simulink model "pipeline_13bit"  (R2022b)
settings: Solver=FixedStepDiscrete  StartTime=0.0  StopTime=5000*ts  FixedStep=ts  RelTol=1e-3
values from neighbouring files (symbols this model uses):
  beta = 1.01    [ADC_13bit.m]
  bits_number = 13    [ADC_13bit.m]
  C = 10e-12    (= 1e-11)    [ADC_13bit.m]
  fin = antismear(fin_pre,fs,nfft)    [ADC_13bit.m]
  Gain = 5000    [ADC_13bit.m]
  k = 1.380649e-23    [ADC_13bit.m]
  T = 300    [ADC_13bit.m]
  ts = 1/fs    (= 1)    [ADC_13bit.m]
(part 3 of 3)

== system pipeline_13bit/SHA_less_13_bit/Subsystem/stage_1p5_bit7/Comparator 2 ==
  Vin : Inport
  Vref : Inport  Port=2
  Output 1 or 0 : Relay  OnSwitchValue=0  OffSwitchValue=0
  Sum : Sum  Inputs=|+-
  Out : Outport
  wires:
  Sum/1 -> Output 1 or 0/1
  Vin/1 -> Sum/1
  Output 1 or 0/1 -> Out/1
  Vref/1 -> Sum/2

== system pipeline_13bit/SHA_less_13_bit/Subsystem/stage_1p5_bit7/Encoder ==
  b1 : Inport
  b2 : Inport  Port=2
  " " : DataTypeConversion  OutDataTypeStr=double  SaturateOnIntegerOverflow=off  RndMeth=Floor
  NOR : Logic  Operator=NOR  AllPortsSameDT=off  OutDataTypeStr=boolean
  NOT : Logic  Operator=NOT  AllPortsSameDT=off  OutDataTypeStr=boolean
  D0 : Outport
  D1 : Outport  Port=2
  wires:
  b2/1 -> NOR/2, D1/1
  NOR/1 -> " "/1
  " "/1 -> D0/1
  NOT/1 -> NOR/1
  b1/1 -> NOT/1

== system pipeline_13bit/SHA_less_13_bit/Subsystem/stage_1p5_bit7/Sub DAC ==
  b1 : Inport
  b2 : Inport  Port=2
  NOT : Logic  Operator=NOT  AllPortsSameDT=off  OutDataTypeStr=boolean
  Subtract : Sum  Inputs=-+
  Vdac : Outport
  wires:
  b2/1 -> Subtract/2
  b1/1 -> NOT/1
  Subtract/1 -> Vdac/1
  NOT/1 -> Subtract/1

== system pipeline_13bit/SHA_less_13_bit/Subsystem/stage_1p5_bit7/Subsystem1 ==
  IN : Inport
  Clock Jitter : Subsystem  Description=Jitter
  Gain : Gain
  Saturation : Saturate  UpperLimit=1000  LowerLimit=-1
  Zero-Order Hold1 : ZeroOrderHold  SampleTime=ts
  S/H : Outport
  wires:
  Zero-Order Hold1/1 -> S/H/1
  Saturation/1 -> Zero-Order Hold1/1
  IN/1 -> Clock Jitter/1(IN)
  Clock Jitter/1(Clock) -> Gain/1
  Gain/1 -> Saturation/1

== system pipeline_13bit/SHA_less_13_bit/Subsystem/stage_1p5_bit8/Comparator 1 ==
  Vin : Inport
  Vref : Inport  Port=2
  Output 1 or 0 : Relay  OnSwitchValue=0  OffSwitchValue=0
  Sum : Sum  Inputs=|+-
  Out : Outport
  wires:
  Sum/1 -> Output 1 or 0/1
  Vin/1 -> Sum/1
  Output 1 or 0/1 -> Out/1
  Vref/1 -> Sum/2

== system pipeline_13bit/SHA_less_13_bit/Subsystem/stage_1p5_bit8/Comparator 2 ==
  Vin : Inport
  Vref : Inport  Port=2
  Output 1 or 0 : Relay  OnSwitchValue=0  OffSwitchValue=0
  Sum : Sum  Inputs=|+-
  Out : Outport
  wires:
  Sum/1 -> Output 1 or 0/1
  Vin/1 -> Sum/1
  Output 1 or 0/1 -> Out/1
  Vref/1 -> Sum/2

== system pipeline_13bit/SHA_less_13_bit/Subsystem/stage_1p5_bit8/Encoder ==
  b1 : Inport
  b2 : Inport  Port=2
  " " : DataTypeConversion  OutDataTypeStr=double  SaturateOnIntegerOverflow=off  RndMeth=Floor
  NOR : Logic  Operator=NOR  AllPortsSameDT=off  OutDataTypeStr=boolean
  NOT : Logic  Operator=NOT  AllPortsSameDT=off  OutDataTypeStr=boolean
  D0 : Outport
  D1 : Outport  Port=2
  wires:
  b2/1 -> NOR/2, D1/1
  NOR/1 -> " "/1
  " "/1 -> D0/1
  NOT/1 -> NOR/1
  b1/1 -> NOT/1

== system pipeline_13bit/SHA_less_13_bit/Subsystem/stage_1p5_bit8/Sub DAC ==
  b1 : Inport
  b2 : Inport  Port=2
  NOT : Logic  Operator=NOT  AllPortsSameDT=off  OutDataTypeStr=boolean
  Subtract : Sum  Inputs=-+
  Vdac : Outport
  wires:
  b2/1 -> Subtract/2
  b1/1 -> NOT/1
  Subtract/1 -> Vdac/1
  NOT/1 -> Subtract/1

== system pipeline_13bit/SHA_less_13_bit/Subsystem/stage_1p5_bit8/Subsystem1 ==
  IN : Inport
  Clock Jitter : Subsystem  Description=Jitter
  Gain : Gain
  Saturation : Saturate  UpperLimit=1000  LowerLimit=-1
  Zero-Order Hold1 : ZeroOrderHold  SampleTime=ts
  S/H : Outport
  wires:
  Zero-Order Hold1/1 -> S/H/1
  Saturation/1 -> Zero-Order Hold1/1
  IN/1 -> Clock Jitter/1(IN)
  Clock Jitter/1(Clock) -> Gain/1
  Gain/1 -> Saturation/1

== system pipeline_13bit/SHA_less_13_bit/Subsystem/stage_3_bit_flash/Comparator 1 ==
  Vin : Inport
  Vref : Inport  Port=2
  Output 1 or 0 : Relay  OnSwitchValue=0  OffSwitchValue=0
  Sum : Sum  Inputs=|+-
  Out : Outport
  wires:
  Sum/1 -> Output 1 or 0/1
  Vin/1 -> Sum/1
  Output 1 or 0/1 -> Out/1
  Vref/1 -> Sum/2

== system pipeline_13bit/SHA_less_13_bit/Subsystem/stage_3_bit_flash/Comparator 2 ==
  Vin : Inport
  Vref : Inport  Port=2
  Output 1 or 0 : Relay  OnSwitchValue=0  OffSwitchValue=0
  Sum : Sum  Inputs=|+-
  Out : Outport
  wires:
  Sum/1 -> Output 1 or 0/1
  Vin/1 -> Sum/1
  Output 1 or 0/1 -> Out/1
  Vref/1 -> Sum/2

== system pipeline_13bit/SHA_less_13_bit/Subsystem/stage_3_bit_flash/Comparator 3 ==
  Vin : Inport
  Vref : Inport  Port=2
  Output 1 or 0 : Relay  OnSwitchValue=0  OffSwitchValue=0
  Sum : Sum  Inputs=|+-
  Out : Outport
  wires:
  Sum/1 -> Output 1 or 0/1
  Vin/1 -> Sum/1
  Output 1 or 0/1 -> Out/1
  Vref/1 -> Sum/2

== system pipeline_13bit/SHA_less_13_bit/Subsystem/stage_3_bit_flash/Comparator 4 ==
  Vin : Inport
  Vref : Inport  Port=2
  Output 1 or 0 : Relay  OnSwitchValue=0  OffSwitchValue=0
  Sum : Sum  Inputs=|+-
  Out : Outport
  wires:
  Sum/1 -> Output 1 or 0/1
  Vin/1 -> Sum/1
  Output 1 or 0/1 -> Out/1
  Vref/1 -> Sum/2

== system pipeline_13bit/SHA_less_13_bit/Subsystem/stage_3_bit_flash/Comparator 5 ==
  Vin : Inport
  Vref : Inport  Port=2
  Output 1 or 0 : Relay  OnSwitchValue=0  OffSwitchValue=0
  Sum : Sum  Inputs=|+-
  Out : Outport
  wires:
  Sum/1 -> Output 1 or 0/1
  Vin/1 -> Sum/1
  Output 1 or 0/1 -> Out/1
  Vref/1 -> Sum/2

== system pipeline_13bit/SHA_less_13_bit/Subsystem/stage_3_bit_flash/Comparator 6 ==
  Vin : Inport
  Vref : Inport  Port=2
  Output 1 or 0 : Relay  OnSwitchValue=0  OffSwitchValue=0
  Sum : Sum  Inputs=|+-
  Out : Outport
  wires:
  Sum/1 -> Output 1 or 0/1
  Vin/1 -> Sum/1
  Output 1 or 0/1 -> Out/1
  Vref/1 -> Sum/2

== system pipeline_13bit/SHA_less_13_bit/Subsystem/stage_3_bit_flash/Comparator 7 ==
  Vin : Inport
  Vref : Inport  Port=2
  Output 1 or 0 : Relay  OnSwitchValue=0  OffSwitchValue=0
  Sum : Sum  Inputs=|+-
  Out : Outport
  wires:
  Sum/1 -> Output 1 or 0/1
  Vin/1 -> Sum/1
  Output 1 or 0/1 -> Out/1
  Vref/1 -> Sum/2

== system pipeline_13bit/SHA_less_13_bit/Subsystem/stage_3_bit_flash/Subsystem1 ==
  IN : Inport
  Clock Jitter : Subsystem  Description=Jitter
  Gain : Gain
  Saturation : Saturate  UpperLimit=1000  LowerLimit=-1
  Zero-Order Hold1 : ZeroOrderHold  SampleTime=ts
  S/H : Outport
  wires:
  Zero-Order Hold1/1 -> S/H/1
  Saturation/1 -> Zero-Order Hold1/1
  IN/1 -> Clock Jitter/1(IN)
  Clock Jitter/1(Clock) -> Gain/1
  Gain/1 -> Saturation/1

== system pipeline_13bit/SHA_less_13_bit/Subsystem/stage_3_bit_flash/Thermometer to Binary Encoder ==
  b1 : Inport
  b2 : Inport  Port=2
  b3 : Inport  Port=3
  b4 : Inport  Port=4
  b5 : Inport  Port=5
  b6 : Inport  Port=6
  b7 : Inport  Port=7
  and{,1..3} (4 alike) : Logic  AllPortsSameDT=off  OutDataTypeStr=boolean
  int1 : DataTypeConversion  OutDataTypeStr=double  SaturateOnIntegerOverflow=off  RndMeth=Floor
  int2 : DataTypeConversion  OutDataTypeStr=double  SaturateOnIntegerOverflow=off  RndMeth=Floor
  int3 : DataTypeConversion  OutDataTypeStr=double  SaturateOnIntegerOverflow=off  RndMeth=Floor
  not : Logic  Operator=NOT  AllPortsSameDT=off  OutDataTypeStr=boolean
  not1 : Logic  Operator=NOT  AllPortsSameDT=off  OutDataTypeStr=boolean
  not2 : Logic  Operator=NOT  AllPortsSameDT=off  OutDataTypeStr=boolean
  or : Logic  Operator=OR  AllPortsSameDT=off  OutDataTypeStr=boolean
  or1 : Logic  Operator=OR  Inputs=4  AllPortsSameDT=off  OutDataTypeStr=boolean
  D0 : Outport
  D1 : Outport  Port=2
  D2 : Outport  Port=3
  wires:
  b4/1 -> not/1, int1/1
  not/1 -> and/2, and2/1
  b2/1 -> and/1, not1/1
  b6/1 -> or/2, not2/1
  and/1 -> or/1
  or/1 -> int2/1
  or1/1 -> int3/1
  b1/1 -> and1/1
  not1/1 -> and1/2
  and1/1 -> or1/1
  b3/1 -> and2/2
  and2/1 -> or1/2
  b7/1 -> or1/4
  not2/1 -> and3/2
  b5/1 -> and3/1
  int2/1 -> D1/1
  int3/1 -> D0/1
  and3/1 -> or1/3
  int1/1 -> D2/1

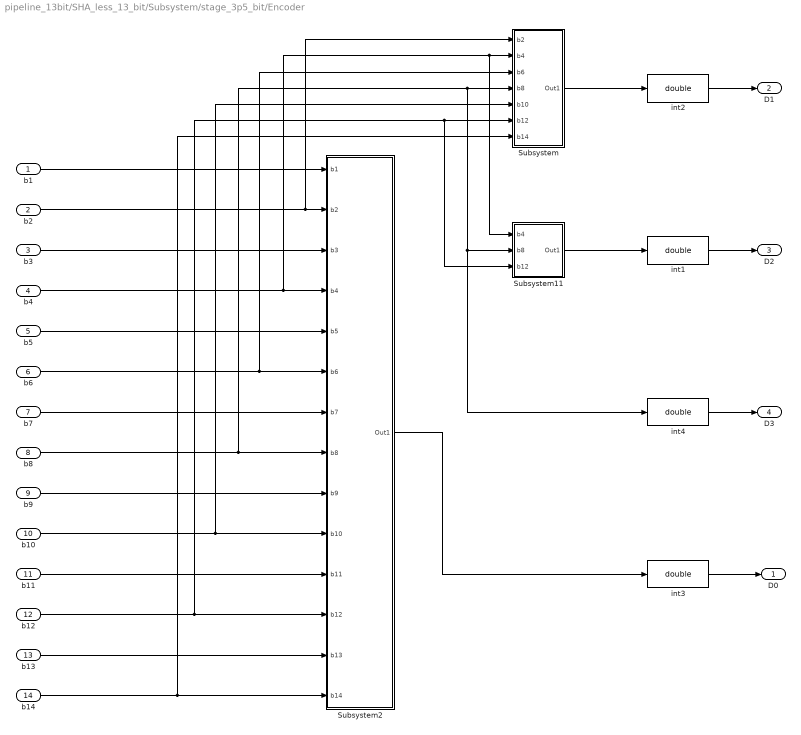
== system pipeline_13bit/SHA_less_13_bit/Subsystem/stage_3p5_bit/Encoder ==
  b1 : Inport
  b2 : Inport  Port=2
  b3 : Inport  Port=3
  b4 : Inport  Port=4
  b5 : Inport  Port=5
  b6 : Inport  Port=6
  b7 : Inport  Port=7
  b8 : Inport  Port=8
  b9 : Inport  Port=9
  b10 : Inport  Port=10
  b11 : Inport  Port=11
  b12 : Inport  Port=12
  b13 : Inport  Port=13
  b14 : Inport  Port=14
  Subsystem : Subsystem
  Subsystem11 : Subsystem
  Subsystem2 : Subsystem
  int{1..4} (4 alike) : DataTypeConversion  OutDataTypeStr=double  SaturateOnIntegerOverflow=off  RndMeth=Floor
  D0 : Outport
  D1 : Outport  Port=2
  D2 : Outport  Port=3
  D3 : Outport  Port=4
  wires:
  int2/1 -> D1/1
  int3/1 -> D0/1
  int1/1 -> D2/1
  int4/1 -> D3/1
  Subsystem11/1(Out1) -> int1/1
  Subsystem/1(Out1) -> int2/1
  Subsystem2/1(Out1) -> int3/1
  b1/1 -> Subsystem2/1(b1)
  b2/1 -> Subsystem/1(b2), Subsystem2/2(b2)
  b3/1 -> Subsystem2/3(b3)
  b4/1 -> Subsystem11/1(b4), Subsystem/2(b4), Subsystem2/4(b4)
  b5/1 -> Subsystem2/5(b5)
  b7/1 -> Subsystem2/7(b7)
  b8/1 -> Subsystem11/2(b8), int4/1, Subsystem/4(b8), Subsystem2/8(b8)
  b9/1 -> Subsystem2/9(b9)
  b10/1 -> Subsystem/5(b10), Subsystem2/10(b10)
  b11/1 -> Subsystem2/11(b11)
  b12/1 -> Subsystem11/3(b12), Subsystem/6(b12), Subsystem2/12(b12)
  b13/1 -> Subsystem2/13(b13)
  b14/1 -> Subsystem/7(b14), Subsystem2/14(b14)
  b6/1 -> Subsystem/3(b6), Subsystem2/6(b6)

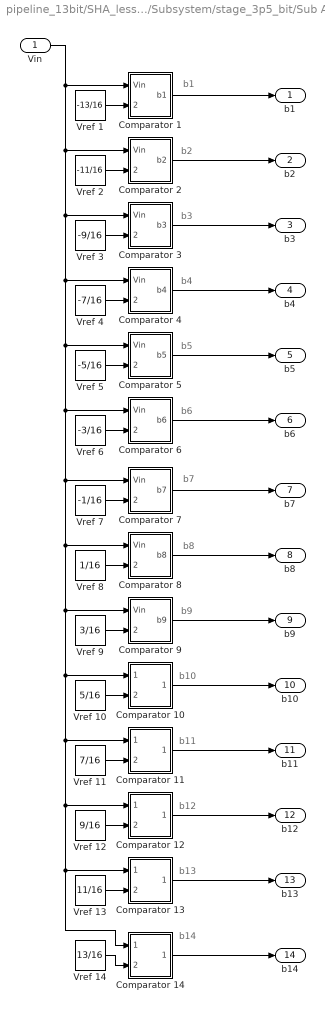
== system pipeline_13bit/SHA_less_13_bit/Subsystem/stage_3p5_bit/Sub ADC ==
  note: b2
  note: b1
  note: b3
  note: b4
  note: b5
  note: b6
  note: b10
  note: b11
  note: b9
  note: b12
  note: b8
  note: b7
  note: b14
  note: b13
  Vin : Inport
  Comparator 1 : Subsystem
  Comparator 10 : Subsystem
  Comparator 11 : Subsystem
  Comparator 12 : Subsystem
  Comparator 13 : Subsystem
  Comparator 14 : Subsystem
  Comparator 2 : Subsystem
  Comparator 3 : Subsystem
  Comparator 4 : Subsystem
  Comparator 5 : Subsystem
  Comparator 6 : Subsystem
  Comparator 7 : Subsystem
  Comparator 8 : Subsystem
  Comparator 9 : Subsystem
  Vref 1 : Constant  Value=-13/16
  Vref 10 : Constant  Value=5/16
  Vref 11 : Constant  Value=7/16
  Vref 12 : Constant  Value=9/16
  Vref 13 : Constant  Value=11/16
  Vref 14 : Constant  Value=13/16
  Vref 2 : Constant  Value=-11/16
  Vref 3 : Constant  Value=-9/16
  Vref 4 : Constant  Value=-7/16
  Vref 5 : Constant  Value=-5/16
  Vref 6 : Constant  Value=-3/16
  Vref 7 : Constant  Value=-1/16
  Vref 8 : Constant  Value=1/16
  Vref 9 : Constant  Value=3/16
  b1 : Outport
  b2 : Outport  Port=2
  b3 : Outport  Port=3
  b4 : Outport  Port=4
  b5 : Outport  Port=5
  b6 : Outport  Port=6
  b7 : Outport  Port=7
  b8 : Outport  Port=8
  b9 : Outport  Port=9
  b10 : Outport  Port=10
  b11 : Outport  Port=11
  b12 : Outport  Port=12
  b13 : Outport  Port=13
  b14 : Outport  Port=14
  wires:
  Vin/1 -> Comparator 1/1(Vin), Comparator 2/1(Vin), Comparator 3/1(Vin), Comparator 4/1(Vin), Comparator 5/1(Vin), Comparator 6/1(Vin), Comparator 7/1(Vin), Comparator 8/1(Vin), Comparator 9/1(Vin), Comparator 10/1(Vin), Comparator 11/1(Vin), Comparator 12/1(Vin), Comparator 13/1(Vin), Comparator 14/1(Vin)
  Vref 1/1 -> Comparator 1/2(Vref)
  Vref 2/1 -> Comparator 2/2(Vref)
  Vref 14/1 -> Comparator 14/2(Vref)
  Vref 4/1 -> Comparator 4/2(Vref)
  Vref 5/1 -> Comparator 5/2(Vref)
  Vref 12/1 -> Comparator 12/2(Vref)
  Comparator 9/1(b9) -> b9/1
  Vref 9/1 -> Comparator 9/2(Vref)
  Comparator 5/1(b5) -> b5/1
  Vref 13/1 -> Comparator 13/2(Vref)
  Vref 6/1 -> Comparator 6/2(Vref)
  Vref 7/1 -> Comparator 7/2(Vref)
  Comparator 2/1(b2) -> b2/1
  Vref 3/1 -> Comparator 3/2(Vref)
  Vref 10/1 -> Comparator 10/2(Vref)
  Comparator 11/1(b11) -> b11/1
  Vref 8/1 -> Comparator 8/2(Vref)
  Vref 11/1 -> Comparator 11/2(Vref)
  Comparator 12/1(b12) -> b12/1
  Comparator 13/1(b13) -> b13/1
  Comparator 10/1(b10) -> b10/1
  Comparator 1/1(b1) -> b1/1
  Comparator 4/1(b4) -> b4/1
  Comparator 8/1(b8) -> b8/1
  Comparator 7/1(b7) -> b7/1
  Comparator 14/1(b14) -> b14/1
  Comparator 3/1(b3) -> b3/1
  Comparator 6/1(b6) -> b6/1

== system pipeline_13bit/SHA_less_13_bit/Subsystem/stage_3p5_bit/Sub DAC ==
  b1 : Inport
  b2 : Inport  Port=2
  b3 : Inport  Port=3
  b4 : Inport  Port=4
  b5 : Inport  Port=5
  b6 : Inport  Port=6
  b7 : Inport  Port=7
  b8 : Inport  Port=8
  b9 : Inport  Port=9
  b10 : Inport  Port=10
  b11 : Inport  Port=11
  b12 : Inport  Port=12
  b13 : Inport  Port=13
  b14 : Inport  Port=14
  Constant : Constant  Value=14
  Gain : Gain  Gain=2
  Gain1 : Gain  Gain=0.5
  Sum : Sum  Inputs=++++++++++++++
  Sum1 : Sum  Inputs=|+-
  Vdac : Outport
  wires:
  Sum/1 -> Gain/1
  Gain/1 -> Sum1/1
  Constant/1 -> Sum1/2
  Sum1/1 -> Gain1/1
  Gain1/1 -> Vdac/1
  b1/1 -> Sum/1
  b2/1 -> Sum/2
  b3/1 -> Sum/3
  b4/1 -> Sum/4
  b5/1 -> Sum/5
  b6/1 -> Sum/6
  b7/1 -> Sum/7
  b8/1 -> Sum/8
  b9/1 -> Sum/9
  b10/1 -> Sum/10
  b11/1 -> Sum/11
  b12/1 -> Sum/12
  b13/1 -> Sum/13
  b14/1 -> Sum/14

== system pipeline_13bit/SHA_less_13_bit/Subsystem/stage_3p5_bit/Subsystem1 ==
  IN : Inport
  Clock Jitter : Subsystem  Description=Jitter
  Gain : Gain
  Saturation : Saturate  UpperLimit=1000  LowerLimit=-1
  Zero-Order Hold1 : ZeroOrderHold  SampleTime=ts
  S/H : Outport
  wires:
  Zero-Order Hold1/1 -> S/H/1
  Saturation/1 -> Zero-Order Hold1/1
  IN/1 -> Clock Jitter/1(IN)
  Clock Jitter/1(Clock) -> Gain/1
  Gain/1 -> Saturation/1

== system pipeline_13bit/13_bit/Subsystem/stage_1p5_bit1/Subsystem1/Clock Jitter ==
  IN : Inport
  Derivative : Derivative
  Product : Product
  Random Number : RandomNumber  SampleTime=ts
  Sum : Sum
  Zero-Order Hold2 : ZeroOrderHold  SampleTime=ts
  Zero-Order Hold3 : ZeroOrderHold  SampleTime=ts
  delta : Gain  Gain=0.02
  Clock : Outport
  wires:
  IN/1 -> Derivative/1, Sum/1
  Product/1 -> Sum/2
  Derivative/1 -> Product/1
  Zero-Order Hold2/1 -> delta/1
  Sum/1 -> Zero-Order Hold3/1
  delta/1 -> Product/2
  Zero-Order Hold3/1 -> Clock/1
  Random Number/1 -> Zero-Order Hold2/1

== system pipeline_13bit/13_bit/Subsystem/stage_1p5_bit2/Subsystem1/Clock Jitter ==
  IN : Inport
  Derivative : Derivative
  Product : Product
  Random Number : RandomNumber  SampleTime=ts
  Sum : Sum
  Zero-Order Hold2 : ZeroOrderHold  SampleTime=ts
  Zero-Order Hold3 : ZeroOrderHold  SampleTime=ts
  delta : Gain  Gain=0.02
  Clock : Outport
  wires:
  IN/1 -> Derivative/1, Sum/1
  Product/1 -> Sum/2
  Derivative/1 -> Product/1
  Zero-Order Hold2/1 -> delta/1
  Sum/1 -> Zero-Order Hold3/1
  delta/1 -> Product/2
  Zero-Order Hold3/1 -> Clock/1
  Random Number/1 -> Zero-Order Hold2/1

== system pipeline_13bit/13_bit/Subsystem/stage_1p5_bit4/Subsystem1/Clock Jitter ==
  IN : Inport
  Derivative : Derivative
  Product : Product
  Random Number : RandomNumber  SampleTime=ts
  Sum : Sum
  Zero-Order Hold2 : ZeroOrderHold  SampleTime=ts
  Zero-Order Hold3 : ZeroOrderHold  SampleTime=ts
  delta : Gain  Gain=0.02
  Clock : Outport
  wires:
  IN/1 -> Derivative/1, Sum/1
  Product/1 -> Sum/2
  Derivative/1 -> Product/1
  Zero-Order Hold2/1 -> delta/1
  Sum/1 -> Zero-Order Hold3/1
  delta/1 -> Product/2
  Zero-Order Hold3/1 -> Clock/1
  Random Number/1 -> Zero-Order Hold2/1

== system pipeline_13bit/13_bit/Subsystem/stage_1p5_bit5/Subsystem1/Clock Jitter ==
  IN : Inport
  Derivative : Derivative
  Product : Product
  Random Number : RandomNumber  SampleTime=ts
  Sum : Sum
  Zero-Order Hold2 : ZeroOrderHold  SampleTime=ts
  Zero-Order Hold3 : ZeroOrderHold  SampleTime=ts
  delta : Gain  Gain=0.02
  Clock : Outport
  wires:
  IN/1 -> Derivative/1, Sum/1
  Product/1 -> Sum/2
  Derivative/1 -> Product/1
  Zero-Order Hold2/1 -> delta/1
  Sum/1 -> Zero-Order Hold3/1
  delta/1 -> Product/2
  Zero-Order Hold3/1 -> Clock/1
  Random Number/1 -> Zero-Order Hold2/1

== system pipeline_13bit/13_bit/Subsystem/stage_1p5_bit6/Subsystem1/Clock Jitter ==
  IN : Inport
  Derivative : Derivative
  Product : Product
  Random Number : RandomNumber  SampleTime=ts
  Sum : Sum
  Zero-Order Hold2 : ZeroOrderHold  SampleTime=ts
  Zero-Order Hold3 : ZeroOrderHold  SampleTime=ts
  delta : Gain  Gain=0.02
  Clock : Outport
  wires:
  IN/1 -> Derivative/1, Sum/1
  Product/1 -> Sum/2
  Derivative/1 -> Product/1
  Zero-Order Hold2/1 -> delta/1
  Sum/1 -> Zero-Order Hold3/1
  delta/1 -> Product/2
  Zero-Order Hold3/1 -> Clock/1
  Random Number/1 -> Zero-Order Hold2/1

== system pipeline_13bit/13_bit/Subsystem/stage_1p5_bit7/Subsystem1/Clock Jitter ==
  IN : Inport
  Derivative : Derivative
  Product : Product
  Random Number : RandomNumber  SampleTime=ts
  Sum : Sum
  Zero-Order Hold2 : ZeroOrderHold  SampleTime=ts
  Zero-Order Hold3 : ZeroOrderHold  SampleTime=ts
  delta : Gain  Gain=0.02
  Clock : Outport
  wires:
  IN/1 -> Derivative/1, Sum/1
  Product/1 -> Sum/2
  Derivative/1 -> Product/1
  Zero-Order Hold2/1 -> delta/1
  Sum/1 -> Zero-Order Hold3/1
  delta/1 -> Product/2
  Zero-Order Hold3/1 -> Clock/1
  Random Number/1 -> Zero-Order Hold2/1

== system pipeline_13bit/13_bit/Subsystem/stage_1p5_bit8/Subsystem1/Clock Jitter ==
  IN : Inport
  Derivative : Derivative
  Product : Product
  Random Number : RandomNumber  SampleTime=ts
  Sum : Sum
  Zero-Order Hold2 : ZeroOrderHold  SampleTime=ts
  Zero-Order Hold3 : ZeroOrderHold  SampleTime=ts
  delta : Gain  Gain=0.02
  Clock : Outport
  wires:
  IN/1 -> Derivative/1, Sum/1
  Product/1 -> Sum/2
  Derivative/1 -> Product/1
  Zero-Order Hold2/1 -> delta/1
  Sum/1 -> Zero-Order Hold3/1
  delta/1 -> Product/2
  Zero-Order Hold3/1 -> Clock/1
  Random Number/1 -> Zero-Order Hold2/1

== system pipeline_13bit/13_bit/Subsystem/stage_3_bit_flash/Subsystem1/Clock Jitter ==
  IN : Inport
  Derivative : Derivative
  Product : Product
  Random Number : RandomNumber  SampleTime=ts
  Sum : Sum
  Zero-Order Hold2 : ZeroOrderHold  SampleTime=ts
  Zero-Order Hold3 : ZeroOrderHold  SampleTime=ts
  delta : Gain  Gain=0.02
  Clock : Outport
  wires:
  IN/1 -> Derivative/1, Sum/1
  Product/1 -> Sum/2
  Derivative/1 -> Product/1
  Zero-Order Hold2/1 -> delta/1
  Sum/1 -> Zero-Order Hold3/1
  delta/1 -> Product/2
  Zero-Order Hold3/1 -> Clock/1
  Random Number/1 -> Zero-Order Hold2/1

== system pipeline_13bit/13_bit/Subsystem/stage_3p5_bit/Encoder/Subsystem ==
  b2 : Inport
  b4 : Inport  Port=2
  b6 : Inport  Port=3
  b8 : Inport  Port=4
  b10 : Inport  Port=5
  b12 : Inport  Port=6
  b14 : Inport  Port=7
  Subsystem2 : Subsystem
  Subsystem3 : Subsystem
  Subsystem4 : Subsystem
  or3 : Logic  Operator=OR  Inputs=4  AllPortsSameDT=off  OutDataTypeStr=boolean
  Out1 : Outport
  wires:
  b8/1 -> Subsystem2/2(b8)
  or3/1 -> Out1/1
  b10/1 -> Subsystem4/1(b10)
  Subsystem3/1(Out1) -> or3/1
  Subsystem4/1(Out1) -> or3/3
  Subsystem2/1(Out1) -> or3/2
  b4/1 -> Subsystem3/2(b4)
  b14/1 -> or3/4
  b12/1 -> Subsystem4/2(b12)
  b6/1 -> Subsystem2/1(b6)
  b2/1 -> Subsystem3/1(b2)

== system pipeline_13bit/13_bit/Subsystem/stage_3p5_bit/Encoder/Subsystem11 ==
  b4 : Inport
  b8 : Inport  Port=2
  b12 : Inport  Port=3
  Subsystem : Subsystem
  or2 : Logic  Operator=OR  AllPortsSameDT=off  OutDataTypeStr=boolean
  Out1 : Outport
  wires:
  b8/1 -> Subsystem/2(b8)
  Subsystem/1(Out1) -> or2/1
  b4/1 -> Subsystem/1(b4)
  or2/1 -> Out1/1
  b12/1 -> or2/2

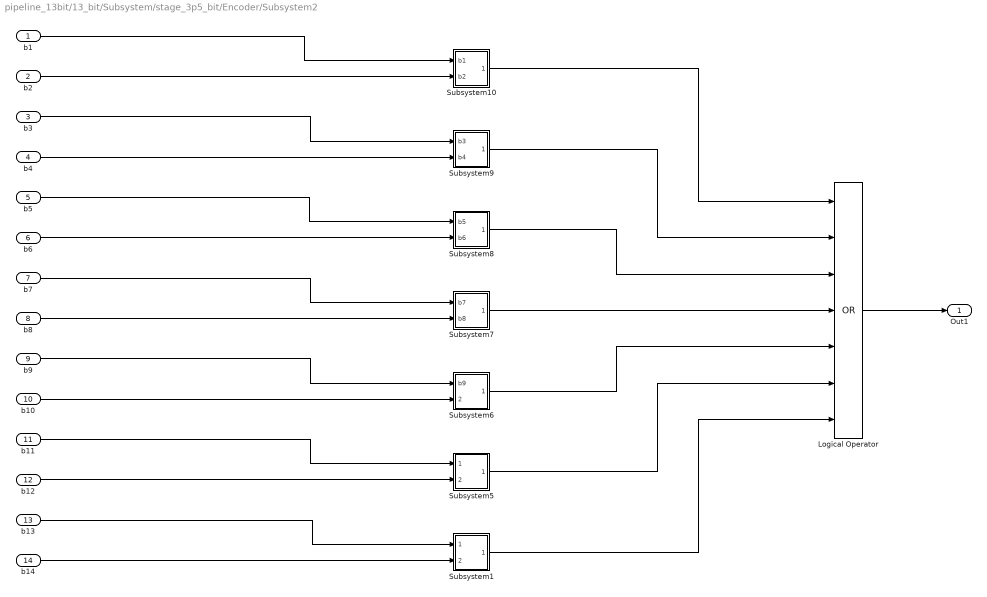
== system pipeline_13bit/13_bit/Subsystem/stage_3p5_bit/Encoder/Subsystem2 ==
  b1 : Inport
  b2 : Inport  Port=2
  b3 : Inport  Port=3
  b4 : Inport  Port=4
  b5 : Inport  Port=5
  b6 : Inport  Port=6
  b7 : Inport  Port=7
  b8 : Inport  Port=8
  b9 : Inport  Port=9
  b10 : Inport  Port=10
  b11 : Inport  Port=11
  b12 : Inport  Port=12
  b13 : Inport  Port=13
  b14 : Inport  Port=14
  Logical Operator : Logic  Operator=OR  Inputs=7  AllPortsSameDT=off  OutDataTypeStr=boolean
  Subsystem1 : Subsystem
  Subsystem10 : Subsystem
  Subsystem5 : Subsystem
  Subsystem6 : Subsystem
  Subsystem7 : Subsystem
  Subsystem8 : Subsystem
  Subsystem9 : Subsystem
  Out1 : Outport
  wires:
  Subsystem7/1(Out1) -> Logical Operator/4
  Subsystem8/1(Out1) -> Logical Operator/3
  Subsystem9/1(Out1) -> Logical Operator/2
  b12/1 -> Subsystem5/2(b12)
  Subsystem6/1(Out1) -> Logical Operator/5
  b14/1 -> Subsystem1/2(b14)
  Subsystem10/1(Out1) -> Logical Operator/1
  Subsystem5/1(Out1) -> Logical Operator/6
  Subsystem1/1(Out1) -> Logical Operator/7
  b7/1 -> Subsystem7/1(b7)
  b6/1 -> Subsystem8/2(b6)
  b8/1 -> Subsystem7/2(b8)
  b10/1 -> Subsystem6/2(b10)
  b5/1 -> Subsystem8/1(b5)
  b11/1 -> Subsystem5/1(b11)
  b2/1 -> Subsystem10/2(b2)
  b4/1 -> Subsystem9/2(b4)
  b3/1 -> Subsystem9/1(b3)
  b9/1 -> Subsystem6/1(b9)
  b1/1 -> Subsystem10/1(b1)
  b13/1 -> Subsystem1/1(b13)
  Logical Operator/1 -> Out1/1

== system pipeline_13bit/13_bit/Subsystem/stage_3p5_bit/Sub ADC/Comparator 1 ==
  Vin : Inport
  Vref : Inport  Port=2
  Output 1 or 0 : Relay  OnSwitchValue=0  OffSwitchValue=0
  Sum : Sum  Inputs=|+-
  b1 : Outport
  wires:
  Sum/1 -> Output 1 or 0/1
  Vin/1 -> Sum/1
  Output 1 or 0/1 -> b1/1
  Vref/1 -> Sum/2

== system pipeline_13bit/13_bit/Subsystem/stage_3p5_bit/Sub ADC/Comparator 10 ==
  Vin : Inport
  Vref : Inport  Port=2
  Output 1 or 0 : Relay  OnSwitchValue=0  OffSwitchValue=0
  Sum : Sum  Inputs=|+-
  b10 : Outport
  wires:
  Sum/1 -> Output 1 or 0/1
  Vin/1 -> Sum/1
  Output 1 or 0/1 -> b10/1
  Vref/1 -> Sum/2

== system pipeline_13bit/13_bit/Subsystem/stage_3p5_bit/Sub ADC/Comparator 11 ==
  Vin : Inport
  Vref : Inport  Port=2
  Output 1 or 0 : Relay  OnSwitchValue=0  OffSwitchValue=0
  Sum : Sum  Inputs=|+-
  b11 : Outport
  wires:
  Sum/1 -> Output 1 or 0/1
  Vin/1 -> Sum/1
  Output 1 or 0/1 -> b11/1
  Vref/1 -> Sum/2

== system pipeline_13bit/13_bit/Subsystem/stage_3p5_bit/Sub ADC/Comparator 12 ==
  Vin : Inport
  Vref : Inport  Port=2
  Output 1 or 0 : Relay  OnSwitchValue=0  OffSwitchValue=0
  Sum : Sum  Inputs=|+-
  b12 : Outport
  wires:
  Sum/1 -> Output 1 or 0/1
  Vin/1 -> Sum/1
  Output 1 or 0/1 -> b12/1
  Vref/1 -> Sum/2

== system pipeline_13bit/13_bit/Subsystem/stage_3p5_bit/Sub ADC/Comparator 13 ==
  Vin : Inport
  Vref : Inport  Port=2
  Output 1 or 0 : Relay  OnSwitchValue=0  OffSwitchValue=0
  Sum : Sum  Inputs=|+-
  b13 : Outport
  wires:
  Sum/1 -> Output 1 or 0/1
  Vin/1 -> Sum/1
  Output 1 or 0/1 -> b13/1
  Vref/1 -> Sum/2

== system pipeline_13bit/13_bit/Subsystem/stage_3p5_bit/Sub ADC/Comparator 14 ==
  Vin : Inport
  Vref : Inport  Port=2
  Output 1 or 0 : Relay  OnSwitchValue=0  OffSwitchValue=0
  Sum : Sum  Inputs=|+-
  b14 : Outport
  wires:
  Sum/1 -> Output 1 or 0/1
  Vin/1 -> Sum/1
  Output 1 or 0/1 -> b14/1
  Vref/1 -> Sum/2

== system pipeline_13bit/13_bit/Subsystem/stage_3p5_bit/Sub ADC/Comparator 2 ==
  Vin : Inport
  Vref : Inport  Port=2
  Output 1 or 0 : Relay  OnSwitchValue=0  OffSwitchValue=0
  Sum : Sum  Inputs=|+-
  b2 : Outport
  wires:
  Sum/1 -> Output 1 or 0/1
  Vin/1 -> Sum/1
  Output 1 or 0/1 -> b2/1
  Vref/1 -> Sum/2

== system pipeline_13bit/13_bit/Subsystem/stage_3p5_bit/Sub ADC/Comparator 3 ==
  Vin : Inport
  Vref : Inport  Port=2
  Output 1 or 0 : Relay  OnSwitchValue=0  OffSwitchValue=0
  Sum : Sum  Inputs=|+-
  b3 : Outport
  wires:
  Sum/1 -> Output 1 or 0/1
  Vin/1 -> Sum/1
  Output 1 or 0/1 -> b3/1
  Vref/1 -> Sum/2

== system pipeline_13bit/13_bit/Subsystem/stage_3p5_bit/Sub ADC/Comparator 4 ==
  Vin : Inport
  Vref : Inport  Port=2
  Output 1 or 0 : Relay  OnSwitchValue=0  OffSwitchValue=0
  Sum : Sum  Inputs=|+-
  b4 : Outport
  wires:
  Sum/1 -> Output 1 or 0/1
  Vin/1 -> Sum/1
  Output 1 or 0/1 -> b4/1
  Vref/1 -> Sum/2

== system pipeline_13bit/13_bit/Subsystem/stage_3p5_bit/Sub ADC/Comparator 5 ==
  Vin : Inport
  Vref : Inport  Port=2
  Output 1 or 0 : Relay  OnSwitchValue=0  OffSwitchValue=0
  Sum : Sum  Inputs=|+-
  b5 : Outport
  wires:
  Sum/1 -> Output 1 or 0/1
  Vin/1 -> Sum/1
  Output 1 or 0/1 -> b5/1
  Vref/1 -> Sum/2

== system pipeline_13bit/13_bit/Subsystem/stage_3p5_bit/Sub ADC/Comparator 6 ==
  Vin : Inport
  Vref : Inport  Port=2
  Output 1 or 0 : Relay  OnSwitchValue=0  OffSwitchValue=0
  Sum : Sum  Inputs=|+-
  b6 : Outport
  wires:
  Sum/1 -> Output 1 or 0/1
  Vin/1 -> Sum/1
  Output 1 or 0/1 -> b6/1
  Vref/1 -> Sum/2

== system pipeline_13bit/13_bit/Subsystem/stage_3p5_bit/Sub ADC/Comparator 7 ==
  Vin : Inport
  Vref : Inport  Port=2
  Output 1 or 0 : Relay  OnSwitchValue=0  OffSwitchValue=0
  Sum : Sum  Inputs=|+-
  b7 : Outport
  wires:
  Sum/1 -> Output 1 or 0/1
  Vin/1 -> Sum/1
  Output 1 or 0/1 -> b7/1
  Vref/1 -> Sum/2

== system pipeline_13bit/13_bit/Subsystem/stage_3p5_bit/Sub ADC/Comparator 8 ==
  Vin : Inport
  Vref : Inport  Port=2
  Output 1 or 0 : Relay  OnSwitchValue=0  OffSwitchValue=0
  Sum : Sum  Inputs=|+-
  b8 : Outport
  wires:
  Sum/1 -> Output 1 or 0/1
  Vin/1 -> Sum/1
  Output 1 or 0/1 -> b8/1
  Vref/1 -> Sum/2

== system pipeline_13bit/13_bit/Subsystem/stage_3p5_bit/Sub ADC/Comparator 9 ==
  Vin : Inport
  Vref : Inport  Port=2
  Output 1 or 0 : Relay  OnSwitchValue=0  OffSwitchValue=0
  Sum : Sum  Inputs=|+-
  b9 : Outport
  wires:
  Sum/1 -> Output 1 or 0/1
  Vin/1 -> Sum/1
  Output 1 or 0/1 -> b9/1
  Vref/1 -> Sum/2

== system pipeline_13bit/13_bit/Subsystem/stage_3p5_bit/Subsystem1/Clock Jitter ==
  IN : Inport
  Derivative : Derivative
  Product : Product
  Random Number : RandomNumber  SampleTime=ts
  Sum : Sum
  Zero-Order Hold2 : ZeroOrderHold  SampleTime=ts
  Zero-Order Hold3 : ZeroOrderHold  SampleTime=ts
  delta : Gain  Gain=0.02
  Clock : Outport
  wires:
  IN/1 -> Derivative/1, Sum/1
  Product/1 -> Sum/2
  Derivative/1 -> Product/1
  Zero-Order Hold2/1 -> delta/1
  Sum/1 -> Zero-Order Hold3/1
  delta/1 -> Product/2
  Zero-Order Hold3/1 -> Clock/1
  Random Number/1 -> Zero-Order Hold2/1

== system pipeline_13bit/SHA_less_13_bit/Subsystem/stage_1p5_bit1/Subsystem1/Clock Jitter ==
  IN : Inport
  Derivative : Derivative
  Product : Product
  Random Number : RandomNumber  SampleTime=ts
  Sum : Sum
  Zero-Order Hold2 : ZeroOrderHold  SampleTime=ts
  Zero-Order Hold3 : ZeroOrderHold  SampleTime=ts
  delta : Gain  Gain=0.02
  Clock : Outport
  wires:
  IN/1 -> Derivative/1, Sum/1
  Product/1 -> Sum/2
  Derivative/1 -> Product/1
  Zero-Order Hold2/1 -> delta/1
  Sum/1 -> Zero-Order Hold3/1
  delta/1 -> Product/2
  Zero-Order Hold3/1 -> Clock/1
  Random Number/1 -> Zero-Order Hold2/1

== system pipeline_13bit/SHA_less_13_bit/Subsystem/stage_1p5_bit2/Subsystem1/Clock Jitter ==
  IN : Inport
  Derivative : Derivative
  Product : Product
  Random Number : RandomNumber  SampleTime=ts
  Sum : Sum
  Zero-Order Hold2 : ZeroOrderHold  SampleTime=ts
  Zero-Order Hold3 : ZeroOrderHold  SampleTime=ts
  delta : Gain  Gain=0.02
  Clock : Outport
  wires:
  IN/1 -> Derivative/1, Sum/1
  Product/1 -> Sum/2
  Derivative/1 -> Product/1
  Zero-Order Hold2/1 -> delta/1
  Sum/1 -> Zero-Order Hold3/1
  delta/1 -> Product/2
  Zero-Order Hold3/1 -> Clock/1
  Random Number/1 -> Zero-Order Hold2/1

== system pipeline_13bit/SHA_less_13_bit/Subsystem/stage_1p5_bit4/Subsystem1/Clock Jitter ==
  IN : Inport
  Derivative : Derivative
  Product : Product
  Random Number : RandomNumber  SampleTime=ts
  Sum : Sum
  Zero-Order Hold2 : ZeroOrderHold  SampleTime=ts
  Zero-Order Hold3 : ZeroOrderHold  SampleTime=ts
  delta : Gain  Gain=0.02
  Clock : Outport
  wires:
  IN/1 -> Derivative/1, Sum/1
  Product/1 -> Sum/2
  Derivative/1 -> Product/1
  Zero-Order Hold2/1 -> delta/1
  Sum/1 -> Zero-Order Hold3/1
  delta/1 -> Product/2
  Zero-Order Hold3/1 -> Clock/1
  Random Number/1 -> Zero-Order Hold2/1

== system pipeline_13bit/SHA_less_13_bit/Subsystem/stage_1p5_bit5/Subsystem1/Clock Jitter ==
  IN : Inport
  Derivative : Derivative
  Product : Product
  Random Number : RandomNumber  SampleTime=ts
  Sum : Sum
  Zero-Order Hold2 : ZeroOrderHold  SampleTime=ts
  Zero-Order Hold3 : ZeroOrderHold  SampleTime=ts
  delta : Gain  Gain=0.02
  Clock : Outport
  wires:
  IN/1 -> Derivative/1, Sum/1
  Product/1 -> Sum/2
  Derivative/1 -> Product/1
  Zero-Order Hold2/1 -> delta/1
  Sum/1 -> Zero-Order Hold3/1
  delta/1 -> Product/2
  Zero-Order Hold3/1 -> Clock/1
  Random Number/1 -> Zero-Order Hold2/1

== system pipeline_13bit/SHA_less_13_bit/Subsystem/stage_1p5_bit6/Subsystem1/Clock Jitter ==
  IN : Inport
  Derivative : Derivative
  Product : Product
  Random Number : RandomNumber  SampleTime=ts
  Sum : Sum
  Zero-Order Hold2 : ZeroOrderHold  SampleTime=ts
  Zero-Order Hold3 : ZeroOrderHold  SampleTime=ts
  delta : Gain  Gain=0.02
  Clock : Outport
  wires:
  IN/1 -> Derivative/1, Sum/1
  Product/1 -> Sum/2
  Derivative/1 -> Product/1
  Zero-Order Hold2/1 -> delta/1
  Sum/1 -> Zero-Order Hold3/1
  delta/1 -> Product/2
  Zero-Order Hold3/1 -> Clock/1
  Random Number/1 -> Zero-Order Hold2/1

== system pipeline_13bit/SHA_less_13_bit/Subsystem/stage_1p5_bit7/Subsystem1/Clock Jitter ==
  IN : Inport
  Derivative : Derivative
  Product : Product
  Random Number : RandomNumber  SampleTime=ts
  Sum : Sum
  Zero-Order Hold2 : ZeroOrderHold  SampleTime=ts
  Zero-Order Hold3 : ZeroOrderHold  SampleTime=ts
  delta : Gain  Gain=0.02
  Clock : Outport
  wires:
  IN/1 -> Derivative/1, Sum/1
  Product/1 -> Sum/2
  Derivative/1 -> Product/1
  Zero-Order Hold2/1 -> delta/1
  Sum/1 -> Zero-Order Hold3/1
  delta/1 -> Product/2
  Zero-Order Hold3/1 -> Clock/1
  Random Number/1 -> Zero-Order Hold2/1

== system pipeline_13bit/SHA_less_13_bit/Subsystem/stage_1p5_bit8/Subsystem1/Clock Jitter ==
  IN : Inport
  Derivative : Derivative
  Product : Product
  Random Number : RandomNumber  SampleTime=ts
  Sum : Sum
  Zero-Order Hold2 : ZeroOrderHold  SampleTime=ts
  Zero-Order Hold3 : ZeroOrderHold  SampleTime=ts
  delta : Gain  Gain=0.02
  Clock : Outport
  wires:
  IN/1 -> Derivative/1, Sum/1
  Product/1 -> Sum/2
  Derivative/1 -> Product/1
  Zero-Order Hold2/1 -> delta/1
  Sum/1 -> Zero-Order Hold3/1
  delta/1 -> Product/2
  Zero-Order Hold3/1 -> Clock/1
  Random Number/1 -> Zero-Order Hold2/1

== system pipeline_13bit/SHA_less_13_bit/Subsystem/stage_3_bit_flash/Subsystem1/Clock Jitter ==
  IN : Inport
  Derivative : Derivative
  Product : Product
  Random Number : RandomNumber  SampleTime=ts
  Sum : Sum
  Zero-Order Hold2 : ZeroOrderHold  SampleTime=ts
  Zero-Order Hold3 : ZeroOrderHold  SampleTime=ts
  delta : Gain  Gain=0.02
  Clock : Outport
  wires:
  IN/1 -> Derivative/1, Sum/1
  Product/1 -> Sum/2
  Derivative/1 -> Product/1
  Zero-Order Hold2/1 -> delta/1
  Sum/1 -> Zero-Order Hold3/1
  delta/1 -> Product/2
  Zero-Order Hold3/1 -> Clock/1
  Random Number/1 -> Zero-Order Hold2/1

== system pipeline_13bit/SHA_less_13_bit/Subsystem/stage_3p5_bit/Encoder/Subsystem ==
  b2 : Inport
  b4 : Inport  Port=2
  b6 : Inport  Port=3
  b8 : Inport  Port=4
  b10 : Inport  Port=5
  b12 : Inport  Port=6
  b14 : Inport  Port=7
  Subsystem2 : Subsystem
  Subsystem3 : Subsystem
  Subsystem4 : Subsystem
  or3 : Logic  Operator=OR  Inputs=4  AllPortsSameDT=off  OutDataTypeStr=boolean
  Out1 : Outport
  wires:
  b8/1 -> Subsystem2/2(b8)
  or3/1 -> Out1/1
  b10/1 -> Subsystem4/1(b10)
  Subsystem3/1(Out1) -> or3/1
  Subsystem4/1(Out1) -> or3/3
  Subsystem2/1(Out1) -> or3/2
  b4/1 -> Subsystem3/2(b4)
  b14/1 -> or3/4
  b12/1 -> Subsystem4/2(b12)
  b6/1 -> Subsystem2/1(b6)
  b2/1 -> Subsystem3/1(b2)

== system pipeline_13bit/SHA_less_13_bit/Subsystem/stage_3p5_bit/Encoder/Subsystem11 ==
  b4 : Inport
  b8 : Inport  Port=2
  b12 : Inport  Port=3
  Subsystem : Subsystem
  or2 : Logic  Operator=OR  AllPortsSameDT=off  OutDataTypeStr=boolean
  Out1 : Outport
  wires:
  b8/1 -> Subsystem/2(b8)
  Subsystem/1(Out1) -> or2/1
  b4/1 -> Subsystem/1(b4)
  or2/1 -> Out1/1
  b12/1 -> or2/2

== system pipeline_13bit/SHA_less_13_bit/Subsystem/stage_3p5_bit/Encoder/Subsystem2 ==
  b1 : Inport
  b2 : Inport  Port=2
  b3 : Inport  Port=3
  b4 : Inport  Port=4
  b5 : Inport  Port=5
  b6 : Inport  Port=6
  b7 : Inport  Port=7
  b8 : Inport  Port=8
  b9 : Inport  Port=9
  b10 : Inport  Port=10
  b11 : Inport  Port=11
  b12 : Inport  Port=12
  b13 : Inport  Port=13
  b14 : Inport  Port=14
  Logical Operator : Logic  Operator=OR  Inputs=7  AllPortsSameDT=off  OutDataTypeStr=boolean
  Subsystem1 : Subsystem
  Subsystem10 : Subsystem
  Subsystem5 : Subsystem
  Subsystem6 : Subsystem
  Subsystem7 : Subsystem
  Subsystem8 : Subsystem
  Subsystem9 : Subsystem
  Out1 : Outport
  wires:
  Subsystem7/1(Out1) -> Logical Operator/4
  Subsystem8/1(Out1) -> Logical Operator/3
  Subsystem9/1(Out1) -> Logical Operator/2
  b12/1 -> Subsystem5/2(b12)
  Subsystem6/1(Out1) -> Logical Operator/5
  b14/1 -> Subsystem1/2(b14)
  Subsystem10/1(Out1) -> Logical Operator/1
  Subsystem5/1(Out1) -> Logical Operator/6
  Subsystem1/1(Out1) -> Logical Operator/7
  b7/1 -> Subsystem7/1(b7)
  b6/1 -> Subsystem8/2(b6)
  b8/1 -> Subsystem7/2(b8)
  b10/1 -> Subsystem6/2(b10)
  b5/1 -> Subsystem8/1(b5)
  b11/1 -> Subsystem5/1(b11)
  b2/1 -> Subsystem10/2(b2)
  b4/1 -> Subsystem9/2(b4)
  b3/1 -> Subsystem9/1(b3)
  b9/1 -> Subsystem6/1(b9)
  b1/1 -> Subsystem10/1(b1)
  b13/1 -> Subsystem1/1(b13)
  Logical Operator/1 -> Out1/1

== system pipeline_13bit/SHA_less_13_bit/Subsystem/stage_3p5_bit/Sub ADC/Comparator 1 ==
  Vin : Inport
  Vref : Inport  Port=2
  Output 1 or 0 : Relay  OnSwitchValue=0  OffSwitchValue=0
  Sum : Sum  Inputs=|+-
  b1 : Outport
  wires:
  Sum/1 -> Output 1 or 0/1
  Vin/1 -> Sum/1
  Output 1 or 0/1 -> b1/1
  Vref/1 -> Sum/2

== system pipeline_13bit/SHA_less_13_bit/Subsystem/stage_3p5_bit/Sub ADC/Comparator 10 ==
  Vin : Inport
  Vref : Inport  Port=2
  Output 1 or 0 : Relay  OnSwitchValue=0  OffSwitchValue=0
  Sum : Sum  Inputs=|+-
  b10 : Outport
  wires:
  Sum/1 -> Output 1 or 0/1
  Vin/1 -> Sum/1
  Output 1 or 0/1 -> b10/1
  Vref/1 -> Sum/2

== system pipeline_13bit/SHA_less_13_bit/Subsystem/stage_3p5_bit/Sub ADC/Comparator 11 ==
  Vin : Inport
  Vref : Inport  Port=2
  Output 1 or 0 : Relay  OnSwitchValue=0  OffSwitchValue=0
  Sum : Sum  Inputs=|+-
  b11 : Outport
  wires:
  Sum/1 -> Output 1 or 0/1
  Vin/1 -> Sum/1
  Output 1 or 0/1 -> b11/1
  Vref/1 -> Sum/2

== system pipeline_13bit/SHA_less_13_bit/Subsystem/stage_3p5_bit/Sub ADC/Comparator 12 ==
  Vin : Inport
  Vref : Inport  Port=2
  Output 1 or 0 : Relay  OnSwitchValue=0  OffSwitchValue=0
  Sum : Sum  Inputs=|+-
  b12 : Outport
  wires:
  Sum/1 -> Output 1 or 0/1
  Vin/1 -> Sum/1
  Output 1 or 0/1 -> b12/1
  Vref/1 -> Sum/2

== system pipeline_13bit/SHA_less_13_bit/Subsystem/stage_3p5_bit/Sub ADC/Comparator 13 ==
  Vin : Inport
  Vref : Inport  Port=2
  Output 1 or 0 : Relay  OnSwitchValue=0  OffSwitchValue=0
  Sum : Sum  Inputs=|+-
  b13 : Outport
  wires:
  Sum/1 -> Output 1 or 0/1
  Vin/1 -> Sum/1
  Output 1 or 0/1 -> b13/1
  Vref/1 -> Sum/2

== system pipeline_13bit/SHA_less_13_bit/Subsystem/stage_3p5_bit/Sub ADC/Comparator 14 ==
  Vin : Inport
  Vref : Inport  Port=2
  Output 1 or 0 : Relay  OnSwitchValue=0  OffSwitchValue=0
  Sum : Sum  Inputs=|+-
  b14 : Outport
  wires:
  Sum/1 -> Output 1 or 0/1
  Vin/1 -> Sum/1
  Output 1 or 0/1 -> b14/1
  Vref/1 -> Sum/2

== system pipeline_13bit/SHA_less_13_bit/Subsystem/stage_3p5_bit/Sub ADC/Comparator 2 ==
  Vin : Inport
  Vref : Inport  Port=2
  Output 1 or 0 : Relay  OnSwitchValue=0  OffSwitchValue=0
  Sum : Sum  Inputs=|+-
  b2 : Outport
  wires:
  Sum/1 -> Output 1 or 0/1
  Vin/1 -> Sum/1
  Output 1 or 0/1 -> b2/1
  Vref/1 -> Sum/2

== system pipeline_13bit/SHA_less_13_bit/Subsystem/stage_3p5_bit/Sub ADC/Comparator 3 ==
  Vin : Inport
  Vref : Inport  Port=2
  Output 1 or 0 : Relay  OnSwitchValue=0  OffSwitchValue=0
  Sum : Sum  Inputs=|+-
  b3 : Outport
  wires:
  Sum/1 -> Output 1 or 0/1
  Vin/1 -> Sum/1
  Output 1 or 0/1 -> b3/1
  Vref/1 -> Sum/2

== system pipeline_13bit/SHA_less_13_bit/Subsystem/stage_3p5_bit/Sub ADC/Comparator 4 ==
  Vin : Inport
  Vref : Inport  Port=2
  Output 1 or 0 : Relay  OnSwitchValue=0  OffSwitchValue=0
  Sum : Sum  Inputs=|+-
  b4 : Outport
  wires:
  Sum/1 -> Output 1 or 0/1
  Vin/1 -> Sum/1
  Output 1 or 0/1 -> b4/1
  Vref/1 -> Sum/2

== system pipeline_13bit/SHA_less_13_bit/Subsystem/stage_3p5_bit/Sub ADC/Comparator 5 ==
  Vin : Inport
  Vref : Inport  Port=2
  Output 1 or 0 : Relay  OnSwitchValue=0  OffSwitchValue=0
  Sum : Sum  Inputs=|+-
  b5 : Outport
  wires:
  Sum/1 -> Output 1 or 0/1
  Vin/1 -> Sum/1
  Output 1 or 0/1 -> b5/1
  Vref/1 -> Sum/2

== system pipeline_13bit/SHA_less_13_bit/Subsystem/stage_3p5_bit/Sub ADC/Comparator 6 ==
  Vin : Inport
  Vref : Inport  Port=2
  Output 1 or 0 : Relay  OnSwitchValue=0  OffSwitchValue=0
  Sum : Sum  Inputs=|+-
  b6 : Outport
  wires:
  Sum/1 -> Output 1 or 0/1
  Vin/1 -> Sum/1
  Output 1 or 0/1 -> b6/1
  Vref/1 -> Sum/2

== system pipeline_13bit/SHA_less_13_bit/Subsystem/stage_3p5_bit/Sub ADC/Comparator 7 ==
  Vin : Inport
  Vref : Inport  Port=2
  Output 1 or 0 : Relay  OnSwitchValue=0  OffSwitchValue=0
  Sum : Sum  Inputs=|+-
  b7 : Outport
  wires:
  Sum/1 -> Output 1 or 0/1
  Vin/1 -> Sum/1
  Output 1 or 0/1 -> b7/1
  Vref/1 -> Sum/2

== system pipeline_13bit/SHA_less_13_bit/Subsystem/stage_3p5_bit/Sub ADC/Comparator 8 ==
  Vin : Inport
  Vref : Inport  Port=2
  Output 1 or 0 : Relay  OnSwitchValue=0  OffSwitchValue=0
  Sum : Sum  Inputs=|+-
  b8 : Outport
  wires:
  Sum/1 -> Output 1 or 0/1
  Vin/1 -> Sum/1
  Output 1 or 0/1 -> b8/1
  Vref/1 -> Sum/2

== system pipeline_13bit/SHA_less_13_bit/Subsystem/stage_3p5_bit/Sub ADC/Comparator 9 ==
  Vin : Inport
  Vref : Inport  Port=2
  Output 1 or 0 : Relay  OnSwitchValue=0  OffSwitchValue=0
  Sum : Sum  Inputs=|+-
  b9 : Outport
  wires:
  Sum/1 -> Output 1 or 0/1
  Vin/1 -> Sum/1
  Output 1 or 0/1 -> b9/1
  Vref/1 -> Sum/2

== system pipeline_13bit/SHA_less_13_bit/Subsystem/stage_3p5_bit/Subsystem1/Clock Jitter ==
  IN : Inport
  Derivative : Derivative
  Product : Product
  Random Number : RandomNumber  SampleTime=ts
  Sum : Sum
  Zero-Order Hold2 : ZeroOrderHold  SampleTime=ts
  Zero-Order Hold3 : ZeroOrderHold  SampleTime=ts
  delta : Gain  Gain=0.02
  Clock : Outport
  wires:
  IN/1 -> Derivative/1, Sum/1
  Product/1 -> Sum/2
  Derivative/1 -> Product/1
  Zero-Order Hold2/1 -> delta/1
  Sum/1 -> Zero-Order Hold3/1
  delta/1 -> Product/2
  Zero-Order Hold3/1 -> Clock/1
  Random Number/1 -> Zero-Order Hold2/1

== system pipeline_13bit/13_bit/Subsystem/stage_3p5_bit/Encoder/Subsystem/Subsystem2 ==
  b6 : Inport
  b8 : Inport  Port=2
  and3 : Logic  AllPortsSameDT=off  OutDataTypeStr=boolean
  not3 : Logic  Operator=NOT  AllPortsSameDT=off  OutDataTypeStr=boolean
  Out1 : Outport
  wires:
  not3/1 -> and3/2
  and3/1 -> Out1/1
  b6/1 -> and3/1
  b8/1 -> not3/1

== system pipeline_13bit/13_bit/Subsystem/stage_3p5_bit/Encoder/Subsystem/Subsystem3 ==
  b2 : Inport
  b4 : Inport  Port=2
  and3 : Logic  AllPortsSameDT=off  OutDataTypeStr=boolean
  not3 : Logic  Operator=NOT  AllPortsSameDT=off  OutDataTypeStr=boolean
  Out1 : Outport
  wires:
  not3/1 -> and3/2
  and3/1 -> Out1/1
  b2/1 -> and3/1
  b4/1 -> not3/1

== system pipeline_13bit/13_bit/Subsystem/stage_3p5_bit/Encoder/Subsystem/Subsystem4 ==
  b10 : Inport
  b12 : Inport  Port=2
  and3 : Logic  AllPortsSameDT=off  OutDataTypeStr=boolean
  not3 : Logic  Operator=NOT  AllPortsSameDT=off  OutDataTypeStr=boolean
  Out1 : Outport
  wires:
  not3/1 -> and3/2
  and3/1 -> Out1/1
  b10/1 -> and3/1
  b12/1 -> not3/1

== system pipeline_13bit/13_bit/Subsystem/stage_3p5_bit/Encoder/Subsystem11/Subsystem ==
  b4 : Inport
  b8 : Inport  Port=2
  and3 : Logic  AllPortsSameDT=off  OutDataTypeStr=boolean
  not3 : Logic  Operator=NOT  AllPortsSameDT=off  OutDataTypeStr=boolean
  Out1 : Outport
  wires:
  not3/1 -> and3/2
  and3/1 -> Out1/1
  b4/1 -> and3/1
  b8/1 -> not3/1

== system pipeline_13bit/13_bit/Subsystem/stage_3p5_bit/Encoder/Subsystem2/Subsystem1 ==
  b13 : Inport
  b14 : Inport  Port=2
  and3 : Logic  AllPortsSameDT=off  OutDataTypeStr=boolean
  not3 : Logic  Operator=NOT  AllPortsSameDT=off  OutDataTypeStr=boolean
  Out1 : Outport
  wires:
  not3/1 -> and3/2
  and3/1 -> Out1/1
  b13/1 -> and3/1
  b14/1 -> not3/1

== system pipeline_13bit/13_bit/Subsystem/stage_3p5_bit/Encoder/Subsystem2/Subsystem10 ==
  b1 : Inport
  b2 : Inport  Port=2
  and3 : Logic  AllPortsSameDT=off  OutDataTypeStr=boolean
  not3 : Logic  Operator=NOT  AllPortsSameDT=off  OutDataTypeStr=boolean
  Out1 : Outport
  wires:
  not3/1 -> and3/2
  and3/1 -> Out1/1
  b1/1 -> and3/1
  b2/1 -> not3/1

== system pipeline_13bit/13_bit/Subsystem/stage_3p5_bit/Encoder/Subsystem2/Subsystem5 ==
  b11 : Inport
  b12 : Inport  Port=2
  and3 : Logic  AllPortsSameDT=off  OutDataTypeStr=boolean
  not3 : Logic  Operator=NOT  AllPortsSameDT=off  OutDataTypeStr=boolean
  Out1 : Outport
  wires:
  not3/1 -> and3/2
  and3/1 -> Out1/1
  b11/1 -> and3/1
  b12/1 -> not3/1

== system pipeline_13bit/13_bit/Subsystem/stage_3p5_bit/Encoder/Subsystem2/Subsystem6 ==
  b9 : Inport
  b10 : Inport  Port=2
  and3 : Logic  AllPortsSameDT=off  OutDataTypeStr=boolean
  not3 : Logic  Operator=NOT  AllPortsSameDT=off  OutDataTypeStr=boolean
  Out1 : Outport
  wires:
  not3/1 -> and3/2
  and3/1 -> Out1/1
  b9/1 -> and3/1
  b10/1 -> not3/1

== system pipeline_13bit/13_bit/Subsystem/stage_3p5_bit/Encoder/Subsystem2/Subsystem7 ==
  b7 : Inport
  b8 : Inport  Port=2
  and3 : Logic  AllPortsSameDT=off  OutDataTypeStr=boolean
  not3 : Logic  Operator=NOT  AllPortsSameDT=off  OutDataTypeStr=boolean
  Out1 : Outport
  wires:
  not3/1 -> and3/2
  and3/1 -> Out1/1
  b7/1 -> and3/1
  b8/1 -> not3/1

== system pipeline_13bit/13_bit/Subsystem/stage_3p5_bit/Encoder/Subsystem2/Subsystem8 ==
  b5 : Inport
  b6 : Inport  Port=2
  and3 : Logic  AllPortsSameDT=off  OutDataTypeStr=boolean
  not3 : Logic  Operator=NOT  AllPortsSameDT=off  OutDataTypeStr=boolean
  Out1 : Outport
  wires:
  not3/1 -> and3/2
  and3/1 -> Out1/1
  b5/1 -> and3/1
  b6/1 -> not3/1

== system pipeline_13bit/13_bit/Subsystem/stage_3p5_bit/Encoder/Subsystem2/Subsystem9 ==
  b3 : Inport
  b4 : Inport  Port=2
  and3 : Logic  AllPortsSameDT=off  OutDataTypeStr=boolean
  not3 : Logic  Operator=NOT  AllPortsSameDT=off  OutDataTypeStr=boolean
  Out1 : Outport
  wires:
  not3/1 -> and3/2
  and3/1 -> Out1/1
  b3/1 -> and3/1
  b4/1 -> not3/1

== system pipeline_13bit/SHA_less_13_bit/Subsystem/stage_3p5_bit/Encoder/Subsystem/Subsystem2 ==
  b6 : Inport
  b8 : Inport  Port=2
  and3 : Logic  AllPortsSameDT=off  OutDataTypeStr=boolean
  not3 : Logic  Operator=NOT  AllPortsSameDT=off  OutDataTypeStr=boolean
  Out1 : Outport
  wires:
  not3/1 -> and3/2
  and3/1 -> Out1/1
  b6/1 -> and3/1
  b8/1 -> not3/1

== system pipeline_13bit/SHA_less_13_bit/Subsystem/stage_3p5_bit/Encoder/Subsystem/Subsystem3 ==
  b2 : Inport
  b4 : Inport  Port=2
  and3 : Logic  AllPortsSameDT=off  OutDataTypeStr=boolean
  not3 : Logic  Operator=NOT  AllPortsSameDT=off  OutDataTypeStr=boolean
  Out1 : Outport
  wires:
  not3/1 -> and3/2
  and3/1 -> Out1/1
  b2/1 -> and3/1
  b4/1 -> not3/1

== system pipeline_13bit/SHA_less_13_bit/Subsystem/stage_3p5_bit/Encoder/Subsystem/Subsystem4 ==
  b10 : Inport
  b12 : Inport  Port=2
  and3 : Logic  AllPortsSameDT=off  OutDataTypeStr=boolean
  not3 : Logic  Operator=NOT  AllPortsSameDT=off  OutDataTypeStr=boolean
  Out1 : Outport
  wires:
  not3/1 -> and3/2
  and3/1 -> Out1/1
  b10/1 -> and3/1
  b12/1 -> not3/1

== system pipeline_13bit/SHA_less_13_bit/Subsystem/stage_3p5_bit/Encoder/Subsystem11/Subsystem ==
  b4 : Inport
  b8 : Inport  Port=2
  and3 : Logic  AllPortsSameDT=off  OutDataTypeStr=boolean
  not3 : Logic  Operator=NOT  AllPortsSameDT=off  OutDataTypeStr=boolean
  Out1 : Outport
  wires:
  not3/1 -> and3/2
  and3/1 -> Out1/1
  b4/1 -> and3/1
  b8/1 -> not3/1

== system pipeline_13bit/SHA_less_13_bit/Subsystem/stage_3p5_bit/Encoder/Subsystem2/Subsystem1 ==
  b13 : Inport
  b14 : Inport  Port=2
  and3 : Logic  AllPortsSameDT=off  OutDataTypeStr=boolean
  not3 : Logic  Operator=NOT  AllPortsSameDT=off  OutDataTypeStr=boolean
  Out1 : Outport
  wires:
  not3/1 -> and3/2
  and3/1 -> Out1/1
  b13/1 -> and3/1
  b14/1 -> not3/1

== system pipeline_13bit/SHA_less_13_bit/Subsystem/stage_3p5_bit/Encoder/Subsystem2/Subsystem10 ==
  b1 : Inport
  b2 : Inport  Port=2
  and3 : Logic  AllPortsSameDT=off  OutDataTypeStr=boolean
  not3 : Logic  Operator=NOT  AllPortsSameDT=off  OutDataTypeStr=boolean
  Out1 : Outport
  wires:
  not3/1 -> and3/2
  and3/1 -> Out1/1
  b1/1 -> and3/1
  b2/1 -> not3/1

== system pipeline_13bit/SHA_less_13_bit/Subsystem/stage_3p5_bit/Encoder/Subsystem2/Subsystem5 ==
  b11 : Inport
  b12 : Inport  Port=2
  and3 : Logic  AllPortsSameDT=off  OutDataTypeStr=boolean
  not3 : Logic  Operator=NOT  AllPortsSameDT=off  OutDataTypeStr=boolean
  Out1 : Outport
  wires:
  not3/1 -> and3/2
  and3/1 -> Out1/1
  b11/1 -> and3/1
  b12/1 -> not3/1

== system pipeline_13bit/SHA_less_13_bit/Subsystem/stage_3p5_bit/Encoder/Subsystem2/Subsystem6 ==
  b9 : Inport
  b10 : Inport  Port=2
  and3 : Logic  AllPortsSameDT=off  OutDataTypeStr=boolean
  not3 : Logic  Operator=NOT  AllPortsSameDT=off  OutDataTypeStr=boolean
  Out1 : Outport
  wires:
  not3/1 -> and3/2
  and3/1 -> Out1/1
  b9/1 -> and3/1
  b10/1 -> not3/1

== system pipeline_13bit/SHA_less_13_bit/Subsystem/stage_3p5_bit/Encoder/Subsystem2/Subsystem7 ==
  b7 : Inport
  b8 : Inport  Port=2
  and3 : Logic  AllPortsSameDT=off  OutDataTypeStr=boolean
  not3 : Logic  Operator=NOT  AllPortsSameDT=off  OutDataTypeStr=boolean
  Out1 : Outport
  wires:
  not3/1 -> and3/2
  and3/1 -> Out1/1
  b7/1 -> and3/1
  b8/1 -> not3/1

== system pipeline_13bit/SHA_less_13_bit/Subsystem/stage_3p5_bit/Encoder/Subsystem2/Subsystem8 ==
  b5 : Inport
  b6 : Inport  Port=2
  and3 : Logic  AllPortsSameDT=off  OutDataTypeStr=boolean
  not3 : Logic  Operator=NOT  AllPortsSameDT=off  OutDataTypeStr=boolean
  Out1 : Outport
  wires:
  not3/1 -> and3/2
  and3/1 -> Out1/1
  b5/1 -> and3/1
  b6/1 -> not3/1

== system pipeline_13bit/SHA_less_13_bit/Subsystem/stage_3p5_bit/Encoder/Subsystem2/Subsystem9 ==
  b3 : Inport
  b4 : Inport  Port=2
  and3 : Logic  AllPortsSameDT=off  OutDataTypeStr=boolean
  not3 : Logic  Operator=NOT  AllPortsSameDT=off  OutDataTypeStr=boolean
  Out1 : Outport
  wires:
  not3/1 -> and3/2
  and3/1 -> Out1/1
  b3/1 -> and3/1
  b4/1 -> not3/1

== matlab function pipeline_13bit/13_bit/Subsystem/Subsystem/GainError/MATLAB Function ==
  data: u input; y output
function y = fcn(u)

y = 1/(1+1/u);

== matlab function pipeline_13bit/13_bit/Subsystem/Subsystem/MATLAB Function ==
  data: u input; y output
function y = fcn(u)

y = u*(1/(2*pi*1.01*5000000)*u+1);
